simulink model "Plant_Model_HT_Cooling_InnerLoop_Harness"  (R2022b)
settings: Solver=VariableStepAuto  StartTime=0.0  StopTime=testdata_input.stack_current(end,1)  RelTol=1e-3
PreLoadFcn:
  | addpath('validation_data\');
InitFcn:
  | load('validation_data\20-07-2023_CTS_Data_to_Feed_Sim.mat')
model workspace: external: MATLAB File C:\Git-Repositories\hctrl_v1_build\hctrl_v1_controller\Plants\h175_model_thermal\Plant_Model_HT_Cooling_Parameters.m (data not in the file)
settings Model: Creator=adrian.taveras  LastModifiedBy=stefan.notter

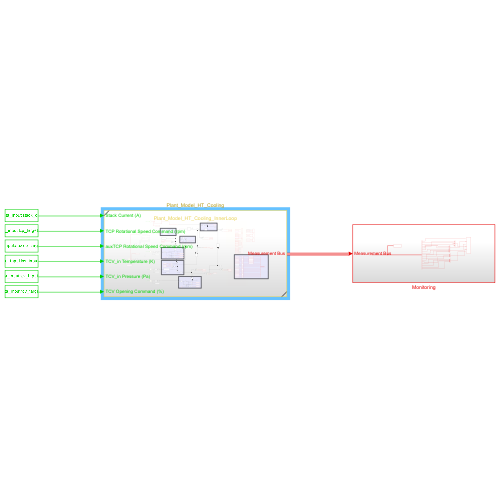
[thumbnail: Simulink's stored preview of the top-level diagram]
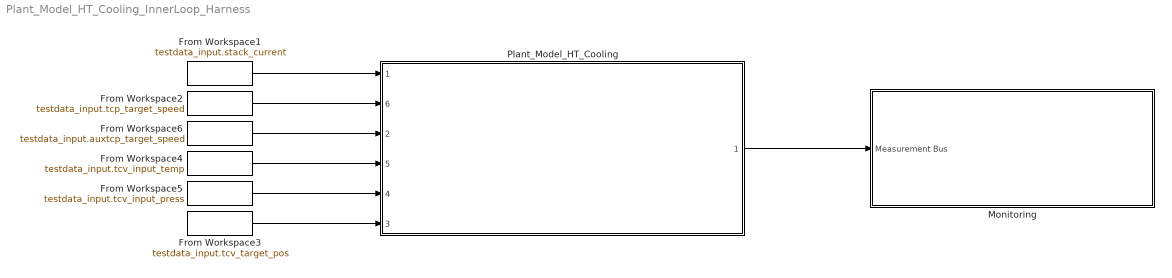
== system Plant_Model_HT_Cooling_InnerLoop_Harness ==
  From Workspace1 : FromWorkspace  VariableName=testdata_input.stack_current  SampleTime=.01
  From Workspace2 : FromWorkspace  VariableName=testdata_input.tcp_target_speed  SampleTime=.01
  From Workspace3 : FromWorkspace  VariableName=testdata_input.tcv_target_pos  SampleTime=.01
  From Workspace4 : FromWorkspace  VariableName=testdata_input.tcv_input_temp  SampleTime=.01
  From Workspace5 : FromWorkspace  VariableName=testdata_input.tcv_input_press  SampleTime=.01
  From Workspace6 : FromWorkspace  VariableName=testdata_input.auxtcp_target_speed  SampleTime=.01
  Monitoring : Subsystem
  Plant_Model_HT_Cooling : Subsystem  ReferencedSubsystem=Plant_Model_HT_Cooling_InnerLoop
      settings: PortSchema="{\"entries\":[{\"content\":{\"sides\":[{\"content\":{\"connectorIds\":[\"Out1\"]},\"type\":\"ConnectorPlacement.EquallySpacedRectSide\",\"uuid\":\"706cf171-be05-45fb-992c-ba5e90f5cdb8\"},{\"content\":{\"connectorIds\":[\"In3\",\"In4\",\"In5\",\"In2\",\"In6\",\"In1\"],\"side\":\"RIGHT\"},\"type\":\"ConnectorPlacement.EquallySpacedRectSide\",\"uuid\":\"bf8ca14f-fef4-4eb5-a927-ccc799898aca\"},{\"content\":{\"connectorIds\":[],\"side\":\"TOP\"},\"type\":\"ConnectorPlacement.EquallySpacedRectSide\",\"uuid\":\"9ad70fe7-ae85-4ea7-9728-0856e6ff40bf\"}]},\"type\":\"ConnectorPlacement.EquallySpacedConnector\",\"uuid\":\"91c985a6-7405-42c3-ac14-8c35e74d3001\"}],\"packageUris\":[\"http://schema.mathworks.com/mf0/Connector/R2020b\"],\"version\":\"1.0\"}"
  wires:
  Plant_Model_HT_Cooling/1 -> Monitoring/1(Measurement Bus)
  From Workspace3/1 -> Plant_Model_HT_Cooling/3
  From Workspace2/1 -> Plant_Model_HT_Cooling/6
  From Workspace1/1 -> Plant_Model_HT_Cooling/1
  From Workspace4/1 -> Plant_Model_HT_Cooling/5
  From Workspace5/1 -> Plant_Model_HT_Cooling/4
  From Workspace6/1 -> Plant_Model_HT_Cooling/2

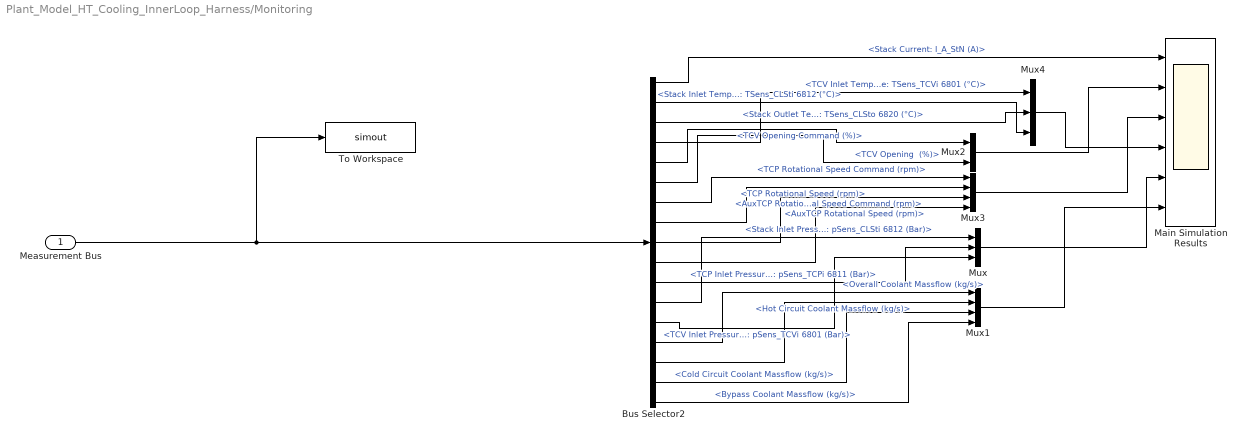
== system Plant_Model_HT_Cooling_InnerLoop_Harness/Monitoring ==
  Measurement Bus : Inport
  Bus Selector2 : BusSelector  OutputSignals="Stack Current: I_A_StN (A),Stack Inlet Temperature: TSens_CLSti 6812 (°C),Stack Outlet Temperature: TSens_CLSto 6820 (°C),TCV Inlet Temperature: TSens_TCVi 6801 (°C),TCV Opening Command (%),TCV Opening  (%),TCP Rotational Speed Command (rpm),TCP Rotational Speed (rpm),AuxTCP Rotational Speed Command (rpm),AuxTCP Rotational Speed (rpm),TCP Inlet Pressure: pSens_TCPi 6811 (Bar),Stack Inlet Pressure: pSens_CLSti 6812 (Bar),TCV Inlet Pressure: pSens_TCVi 6801 (Bar),Overall Coolant Massflow (kg/s),Hot Circuit Coolant Massflow (kg/s),Cold Circuit Coolant Massflow (kg/s),Bypass Coolant Massflow (kg/s)"
  Main Simulation Results : Scope  NumInputPorts=6
  Mux : Mux  Inputs=3
  Mux1 : Mux
  Mux2 : Mux  Inputs=2
  Mux3 : Mux
  Mux4 : Mux  Inputs=3
  To Workspace : ToWorkspace  VariableName=simout  SaveFormat=Timeseries  SampleTime=-1
  wires:
  Bus Selector2/10 -> Mux3/4  "<AuxTCP Rotational Speed (rpm)>"
  Mux4/1 -> Main Simulation Results/4
  Bus Selector2/11 -> Mux/2  "<TCP Inlet Pressure: pSens_TCPi 6811 (Bar)>"
  Mux3/1 -> Main Simulation Results/3
  Bus Selector2/7 -> Mux3/1  "<TCP Rotational Speed Command (rpm)>"
  Bus Selector2/3 -> Mux4/2  "<Stack Outlet Temperature: TSens_CLSto 6820 (°C)>"
  Mux2/1 -> Main Simulation Results/2
  Measurement Bus/1 -> To Workspace/1, Bus Selector2/1
  Bus Selector2/9 -> Mux3/3  "<AuxTCP Rotational Speed Command (rpm)>"
  Bus Selector2/2 -> Mux4/3  "<Stack Inlet Temperature: TSens_CLSti 6812 (°C)>"
  Bus Selector2/6 -> Mux2/2  "<TCV Opening  (%)>"
  Mux/1 -> Main Simulation Results/5
  Bus Selector2/15 -> Mux1/2  "<Hot Circuit Coolant Massflow (kg/s)>"
  Bus Selector2/13 -> Mux/3  "<TCV Inlet Pressure: pSens_TCVi 6801 (Bar)>"
  Bus Selector2/14 -> Mux1/1  "<Overall Coolant Massflow (kg/s)>"
  Mux1/1 -> Main Simulation Results/6
  Bus Selector2/17 -> Mux1/4  "<Bypass Coolant Massflow (kg/s)>"
  Bus Selector2/8 -> Mux3/2  "<TCP Rotational Speed (rpm)>"
  Bus Selector2/5 -> Mux2/1  "<TCV Opening Command (%)>"
  Bus Selector2/16 -> Mux1/3  "<Cold Circuit Coolant Massflow (kg/s)>"
  Bus Selector2/12 -> Mux/1  "<Stack Inlet Pressure: pSens_CLSti 6812 (Bar)>"
  Bus Selector2/1 -> Main Simulation Results/1  "<Stack Current: I_A_StN (A)>"
  Bus Selector2/4 -> Mux4/1  "<TCV Inlet Temperature: TSens_TCVi 6801 (°C)>"
